simulink model "Primero"  (R2017b)
settings: Solver=VariableStepAuto  StartTime=0.0  StopTime=3  RelTol=1e-3
settings Model: Creator=Cx001la  LastModifiedBy=Cx001la

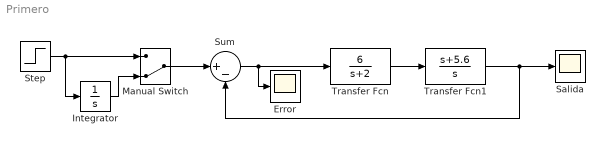
== system Primero ==
  Error : Scope
  Integrator : Integrator
  Manual Switch : ManualSwitch  CurrentSetting=0
  Salida : Scope
  Step : Step  Time=0  SampleTime=0
  Sum : Sum  Inputs=|+-
  Transfer Fcn : TransferFcn  Numerator=[6]  Denominator=[1 2]
  Transfer Fcn1 : TransferFcn  Numerator=[1 5.6]  Denominator=[1 0]
  wires:
  Transfer Fcn/1 -> Transfer Fcn1/1
  Sum/1 -> Error/1, Transfer Fcn/1
  Transfer Fcn1/1 -> Salida/1, Sum/2
  Integrator/1 -> Manual Switch/2
  Manual Switch/1 -> Sum/1
  Step/1 -> Integrator/1, Manual Switch/1
